simulink model "part2_MAIN"  (R2023b)
settings: Solver=FixedStepAuto  StartTime=0.0  StopTime=300  FixedStep=0.1  RelTol=1e-3
values from neighbouring files (symbols this model uses):
  Af = diag(ti)    [init.m]
  Aw = [zeros(3) eye(3) ... (first row only)    [get_observer_parameters.m]
  B = [zeros(6,3);zeros(3,3);zeros(3,3);inv(M)]    [get_observer_parameters.m]
  change_position_time = 1200    [init.m]
  Cw = [zeros(3) eye(3)]    [get_observer_parameters.m]
  D = Damping    [init.m]
  Damping = diag([2.6486e5, 8.8164e5, 3.3774e8])    [init.m]
  direction_limit = pi/36    (= 0.0872664625997)    [init.m]
  direction_time_constant = 100    [init.m]
  dt = 0.1    [get_observer_parameters.m]
  E = [Ew, zeros(6,3) ... (first row only)    [get_observer_parameters.m]
  Gamma = diag(omega_is)    [init.m]
  gust_limit = 40    [init.m]
  H = [Cw, eye(3), zeros(3,3) zeros(3,3)]    [get_observer_parameters.m]
  height = 3    [init.m]
  inv_M = inv(M)    [get_observer_parameters.m]
  inv_Tb = inv(Tb)    [get_observer_parameters.m]
  kappa = 0.003    [init.m]
  kappa2 = 0.0026    [init.m]
  Kd = [1660451.40544401; 3920391.80535684; 1605063439.04156]    [init.m]
  Ki = [137.081306245593; 3163.274947400198; 335358.448218978]    [init.m]
  Kp = [75459.3345349083; 277551.73586971; 120744473.878042]    [init.m]
  L = 1800    [init.m]
  M = Mass    [init.m]
  mean_wind_direction = pi    (= 3.14159265359)    [init.m]
  observer_type = 0    [init.m]
  Omega = diag([omega_n])    [get_observer_parameters.m]    (also in init.m = diag(2*omega_is.*zeta_is))
  Q = diag([0.1,0.1,pi/180,1e6,1e6,1e9])*10e3    [get_observer_parameters.m]
  R = diag([0.00001,0.00001,0.01*pi/180])*10e-4    [get_observer_parameters.m]
  simu_step = 36    [init.m]
  simulation = 5    [init.m]
  slow_varying_limit = 1    [init.m]
  slow_varying_time_constant = 100    [init.m]
  TAU = dt*E    [get_observer_parameters.m]
  Tb = 0.1 * eye(3)    [get_observer_parameters.m]
  thruster_type = 0    [init.m]
  u10 = 12    [init.m]
  wind = 1    [init.m]
  x_current = u_c*cos(xi)    [init.m]
  y_current = u_c*sin(xi)    [init.m]
undefined symbols (not defined in the file or in its folder): Hoerner, ModelParams, npf, Param, thrusters, vessel, WaveModel
libraries: dspsigops x42, simulink x30, marine_hydro x16, marine_gnc x8, slpidlib x3
(part 3 of 8)

== system part2_MAIN/Simulation 4/Wave ==
  eta : Inport
  waves : Inport  Port=2
  Gain : Gain  Gain=waveforces
  Sum : Sum
  Wave loads (U=0) : marine_hydro/Hydro Library/Wave loads (U=0)  SystemSampleTime=-1  VariantActivationTime=update diagram  AllowFlexibleInterface=on  Latency=0  AutoFrameSizeCalculation=off
  Wave : Outport  VectorParamsAs1DForOutWhenUnconnected=off
  wires:
  eta/1 -> Wave loads (U=0)/1
  waves/1 -> Wave loads (U=0)/2
  Sum/1 -> Gain/1
  Wave loads (U=0)/1 -> Sum/1
  Wave loads (U=0)/2 -> Sum/2
  Gain/1 -> Wave/1

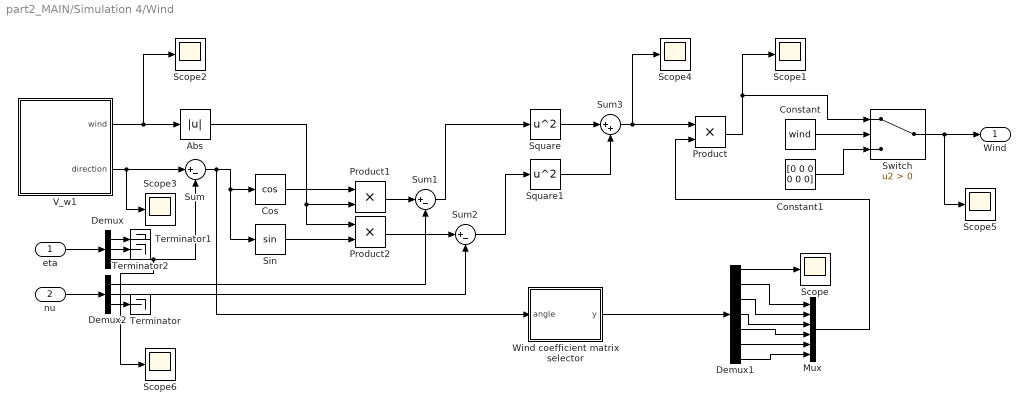
== system part2_MAIN/Simulation 4/Wind ==
  eta : Inport
  nu : Inport  Port=2
  Abs : Abs  SaturateOnIntegerOverflow=off
  Constant : Constant  Value=wind
  Constant1 : Constant  Value=[0 0 0 0 0 0]
  Cos : Trigonometry  Operator=cos
  Demux : Demux  Outputs=3
  Demux1 : Demux  Outputs=7
  Demux2 : Demux  Outputs=3
  Mux : Mux  Inputs=6
  Product : Product
  Product1 : Product
  Product2 : Product
  Scope{,1..6} (7 alike) : Scope
  Sin : Trigonometry
  Square : Math  Operator=square  SignedPower=on
  Square1 : Math  Operator=square  SignedPower=on
  Sum : Sum  Inputs=|+-
  Sum1 : Sum  Inputs=|+-
  Sum2 : Sum  Inputs=|+-
  Sum3 : Sum  Inputs=|++
  Switch : Switch  Criteria=u2 > Threshold  SaturateOnIntegerOverflow=off  InputSameDT=off
  Terminator : Terminator
  Terminator1 : Terminator
  Terminator2 : Terminator
  V_w1 : Subsystem
  Wind coefficient matrix selector : MATLAB Function  TreatAsAtomicUnit=on
  Wind : Outport  VectorParamsAs1DForOutWhenUnconnected=off
  wires:
  V_w1/1(wind) -> Scope2/1, Abs/1
  Abs/1 -> Product2/1, Product1/2
  eta/1 -> Demux/1
  V_w1/2(direction) -> Scope3/1, Sum/1
  Demux/3 -> Scope6/1, Sum/2
  Wind coefficient matrix selector/1(y) -> Demux1/1
  Demux1/1 -> Scope/1
  Demux1/2 -> Mux/1
  Demux1/3 -> Mux/2
  Demux1/4 -> Mux/3
  Demux1/5 -> Mux/4
  Demux1/6 -> Mux/5
  Demux1/7 -> Mux/6
  Product/1 -> Switch/1, Scope1/1
  Mux/1 -> Product/2
  Sum/1 -> Wind coefficient matrix selector/1(angle), Sin/1, Cos/1
  nu/1 -> Demux2/1
  Sin/1 -> Product2/2
  Cos/1 -> Product1/1
  Product1/1 -> Sum1/1
  Product2/1 -> Sum2/1
  Demux2/1 -> Sum1/2
  Demux2/2 -> Sum2/2
  Sum1/1 -> Square/1
  Sum2/1 -> Square1/1
  Sum3/1 -> Scope4/1, Product/1
  Square/1 -> Sum3/1
  Square1/1 -> Sum3/2
  Demux2/3 -> Terminator/1
  Demux/1 -> Terminator1/1
  Demux/2 -> Terminator2/1
  Switch/1 -> Scope5/1, Wind/1
  Constant/1 -> Switch/2
  Constant1/1 -> Switch/3

== system part2_MAIN/Simulation 5/Current (North - East) ==
  note: simulation 2
  note: simulation 1
  eta : Inport
  Constant : Constant
  Constant1 : Constant  Value=[0.5*cos(135); 0.5*sin(135); 0]
  Demux : Demux  Outputs=3
  MATLAB Function : MATLAB Function  TreatAsAtomicUnit=on
  Matrix Multiply : Product  Multiplication=Matrix(*)
  Mux : Mux
  Scope : Scope  NumInputPorts=2
  Scope1 : Scope
  Step : Step  After=0  SampleTime=0
  Subsystem : Subsystem
  Subsystem1 : Subsystem
  Subsystem2 : Subsystem
  Switch : Switch  Criteria=u2 > Threshold  Threshold=1  SaturateOnIntegerOverflow=off  InputSameDT=off
  Switch1 : Switch  Criteria=u2 > Threshold  Threshold=2  SaturateOnIntegerOverflow=off  InputSameDT=off
  Terminator : Terminator
  Terminator1 : Terminator
  Terminator2 : Terminator
  To Workspace : ToWorkspace  VariableName=Current  SaveFormat=Timeseries  SampleTime=-1
  Current1 : Outport  VectorParamsAs1DForOutWhenUnconnected=off
  wires:
  Demux/2 -> Terminator1/1
  MATLAB Function/1(y) -> Matrix Multiply/1
  Switch/1 -> Switch1/3
  Matrix Multiply/1 -> Scope/2, Mux/1
  Subsystem2/1(Out1) -> Switch1/1
  Subsystem/1(Out1) -> Switch/3
  Subsystem1/1(Out1) -> Switch/1
  Demux/1 -> Terminator/1
  Switch1/1 -> Scope/1, To Workspace/1, Matrix Multiply/2
  eta/1 -> Demux/1  "eta"
  Constant/1 -> Switch1/2, Switch/2
  Constant1/1 -> Terminator2/1
  Step/1 -> Mux/3, Mux/2, Mux/4
  Demux/3 -> MATLAB Function/1(u)
  Mux/1 -> Scope1/1, Current1/1

== system part2_MAIN/Simulation 5/DP Controller ==
  note: PID controller
  note: Velocity
  note: Position
  nu : Inport
  eta : Inport  Port=2
  eta set point : Inport  Port=3
  nu setpoint : Inport  Port=4
  Add : Sum  Inputs=+++
  Constant : Constant  Value=0
  Demux{,1,3..4} (4 alike) : Demux  Outputs=3
  Gain : Gain  Gain=Kd
  Gain1 : Gain  Gain=Kp
  Gain2 : Gain  Gain=Ki
  Integrator : Integrator
  MATLAB Function : MATLAB Function  TreatAsAtomicUnit=on
  MATLAB Function1 : MATLAB Function  TreatAsAtomicUnit=on
  Matrix Multiply : Product  Multiplication=Matrix(*)
  Matrix Multiply1 : Product  Multiplication=Matrix(*)
  Mux : Mux  Inputs=3
  Mux2 : Mux  Inputs=6
  Mux3 : Mux  Inputs=3
  Scope : Scope
  Step : Step  After=0  SampleTime=0
  Sum{,1..3} (4 alike) : Sum  Inputs=|-+
  Terminator1 : Terminator
  To Workspace : ToWorkspace  VariableName=simout2  SaveFormat=Timeseries  SampleTime=-1
  tau (body frame) : Outport  VectorParamsAs1DForOutWhenUnconnected=off
  wires:
  eta/1 -> Demux/1  "eta"
  eta set point/1 -> Demux1/1
  Demux/1 -> Sum2/1  "n_vessel"
  Demux1/1 -> Sum2/2  "n_sp"
  Demux/2 -> Sum/1  "e_vessel"
  Demux1/2 -> Sum/2  "e_sp"
  Sum2/1 -> Mux/1
  Sum/1 -> Mux/2
  MATLAB Function/1(y) -> Matrix Multiply/1
  Mux/1 -> Matrix Multiply/2  "error NED frame"
  Step/1 -> Mux2/4, Mux2/3, Mux2/5
  Demux1/3 -> Sum1/2, MATLAB Function1/1(u)  "yaw_sp"
  Sum1/1 -> Mux3/3
  Constant/1 -> Mux/3
  Demux/3 -> MATLAB Function/1(u), Sum1/1  "yaw_vessel"
  Matrix Multiply/1 -> Demux4/1  "error body frame"
  nu/1 -> Sum3/1
  Sum3/1 -> Gain/1  "error body frame"
  nu setpoint/1 -> Matrix Multiply1/2
  MATLAB Function1/1(y) -> Matrix Multiply1/1
  Matrix Multiply1/1 -> Sum3/2
  Integrator/1 -> Gain2/1
  Gain1/1 -> Add/1
  Gain2/1 -> Add/2
  Gain/1 -> Add/3
  Demux3/1 -> Mux2/1
  Demux3/2 -> Mux2/2
  Demux3/3 -> Mux2/6
  Demux4/1 -> Mux3/1
  Demux4/2 -> Mux3/2
  Demux4/3 -> Terminator1/1
  Mux3/1 -> Integrator/1, Gain1/1
  Mux2/1 -> tau (body frame)/1
  Add/1 -> To Workspace/1, Scope/1, Demux3/1

== system part2_MAIN/Simulation 5/Observer ==
  y : Inport
  tau_est : Inport  Port=2
  Demux : Demux  Outputs=2
  EKF : Subsystem
  Memory : Memory  InitialCondition=zeros(3,1)
  Memory2 : Memory  InitialCondition=zeros(3,1)
  Mux : Mux  Inputs=2
  Mux1 : Mux  Inputs=2
  Observer Selector : Constant  Value=observer_type
  Passive Non-Linear : Subsystem
  Subsystem : Subsystem
  Switch : Switch  Criteria=u2 > Threshold  SaturateOnIntegerOverflow=off  InputSameDT=off
  nu_hat : Outport  VectorParamsAs1DForOutWhenUnconnected=off
  eta_hat : Outport  Port=2  VectorParamsAs1DForOutWhenUnconnected=off
  wires:
  tau_est/1 -> Subsystem/1(In1)
  Memory/1 -> EKF/2(U)
  Subsystem/1(Out1) -> Memory/1, Memory2/1
  EKF/1(eta_hat) -> Mux/1
  EKF/2(nu_hat) -> Mux/2
  Passive Non-Linear/1(eta_hat) -> Mux1/1
  Passive Non-Linear/2(nu_hat) -> Mux1/2
  Mux1/1 -> Switch/1
  Observer Selector/1 -> Switch/2
  Mux/1 -> Switch/3
  Switch/1 -> Demux/1
  Demux/1 -> eta_hat/1
  Demux/2 -> nu_hat/1
  y/1 -> EKF/1(y), Passive Non-Linear/1(y)
  Memory2/1 -> Passive Non-Linear/2(tau_est)

== system part2_MAIN/Simulation 5/Reference Model ==
  note: Af
  note: eta_r
  note: Xref
  note: omega
  note: eta_r - Xref
  note: Gamma
  note: x_ddot
  note: Gamma
  note: X_dot
  note: X
  Add : Sum  Inputs=+--
  Gain : Gain  Gain=Af  Multiplication=Matrix(K*u)
  Gain1 : Gain  Gain=Gamma  Multiplication=Matrix(K*u)
  Gain2 : Gain  Gain=Omega  Multiplication=Matrix(K*u)
  Gain3 : Gain  Gain=Gamma  Multiplication=Matrix(K*u)
  Integrator : Integrator
  Integrator1 : Integrator
  Integrator2 : Integrator
  Scope : Scope  NumInputPorts=2
  Scope1 : Scope
  Scope2 : Scope
  Simulation Selector : Subsystem
  Sum : Sum  Inputs=|+-
  To Workspace : ToWorkspace  VariableName=Reference  SaveFormat=Timeseries  SampleTime=-1
  Set-point : Outport  VectorParamsAs1DForOutWhenUnconnected=off
  nu set point : Outport  Port=2  VectorParamsAs1DForOutWhenUnconnected=off
  wires:
  Integrator/1 -> Gain1/1, Sum/2
  Add/1 -> Scope2/1, Integrator1/1
  Integrator2/1 -> To Workspace/1, Scope/1, Set-point/1, Gain3/1
  Gain1/1 -> Add/1
  Integrator1/1 -> nu set point/1, Scope/2, Integrator2/1, Gain2/1
  Gain/1 -> Integrator/1
  Gain2/1 -> Add/3
  Gain3/1 -> Add/2
  Simulation Selector/1(Out1) -> Scope1/1, Sum/1
  Sum/1 -> Gain/1

== system part2_MAIN/Simulation 5/Thrust Allocation ==
  tau_d : Inport
  0 : MATLAB Function  TreatAsAtomicUnit=on
  1 : MATLAB Function  Commented=on  TreatAsAtomicUnit=on
  Constant : Constant  Value=thruster_type
  Switch : Switch  Criteria=u2 > Threshold  SaturateOnIntegerOverflow=off  InputSameDT=off
  Switch1 : Switch  Criteria=u2 > Threshold  SaturateOnIntegerOverflow=off  InputSameDT=off
  Unwrap : Subsystem
  Unwrap1 : Subsystem
  u : Outport  VectorParamsAs1DForOutWhenUnconnected=off
  alpha [rad] : Outport  Port=2  VectorParamsAs1DForOutWhenUnconnected=off
  wires:
  tau_d/1 -> 1/1(tau_d), 0/1(tau_d)
  1/2(alpha) -> Unwrap/1(alpha)
  0/2(alpha) -> Unwrap1/1(alpha)
  1/1(Td) -> Switch/1
  Constant/1 -> Switch1/2, Switch/2
  0/1(Td) -> Switch/3
  Unwrap/1(alpha [rad]) -> Switch1/1
  Unwrap1/1(alpha [rad]) -> Switch1/3
  Switch/1 -> u/1
  Switch1/1 -> alpha [rad]/1

== system part2_MAIN/Simulation 5/Thruster Dynamics ==
  u [N] : Inport
  alpha [rad] : Inport  Port=2
  Constant : Constant  Value=[thrusters(1).xposition, thrusters(2).xposition, thrusters(3).xposition, thrusters(4).xposition, thrusters(5).xposition]
  Constant1 : Constant  Value=zeros(3,1)
  Constant2 : Constant  Value=[thrusters(1).yposition, thrusters(2).yposition, thrusters(3).yposition, thrusters(4).yposition, thrusters(5).yposition]
  Demux : Demux  Outputs=5
  Demux1 : Demux  Outputs=5
  Gain1 : Gain  Gain=1-thrusterfault
  Gain2 : Gain  Gain=1-thrusterfault
  MATLAB Function : MATLAB Function  TreatAsAtomicUnit=on
  Mux1 : Mux  Inputs=2
  Rate Limiter : RateLimiter  RisingSlewLimit=thrusters(1).rate  FallingSlewLimit=-thrusters(1).rate  SampleTimeMode=inherited
  Rate Limiter1 : RateLimiter  RisingSlewLimit=thrusters(2).rate  FallingSlewLimit=-thrusters(2).rate  SampleTimeMode=inherited
  Rate Limiter10 : RateLimiter  RisingSlewLimit=thrusters(4).rotationspeed  FallingSlewLimit=-thrusters(4).rotationspeed  SampleTimeMode=inherited
  Rate Limiter11 : RateLimiter  RisingSlewLimit=thrusters(5).rotationspeed  FallingSlewLimit=-thrusters(5).rotationspeed  SampleTimeMode=inherited
  Rate Limiter2 : RateLimiter  RisingSlewLimit=thrusters(3).rate  FallingSlewLimit=-thrusters(3).rate  SampleTimeMode=inherited
  Rate Limiter4 : RateLimiter  RisingSlewLimit=thrusters(4).rate  FallingSlewLimit=-thrusters(4).rate  SampleTimeMode=inherited
  Rate Limiter5 : RateLimiter  RisingSlewLimit=thrusters(5).rate  FallingSlewLimit=-thrusters(5).rate  SampleTimeMode=inherited
  Rate Limiter8 : RateLimiter  RisingSlewLimit=thrusters(2).rotationspeed  FallingSlewLimit=-thrusters(2).rotationspeed  SampleTimeMode=inherited
  Saturation : Saturate  UpperLimit=thrusters(1).thrust  LowerLimit=-thrusters(1).thrust
  Saturation1 : Saturate  UpperLimit=thrusters(2).thrust  LowerLimit=-thrusters(2).thrust
  Saturation2 : Saturate  UpperLimit=thrusters(3).thrust  LowerLimit=-thrusters(3).thrust
  Saturation4 : Saturate  UpperLimit=thrusters(4).thrust  LowerLimit=-thrusters(4).thrust
  Saturation5 : Saturate  UpperLimit=thrusters(5).thrust  LowerLimit=-thrusters(5).thrust
  Selector4 : Selector  InputPortWidth=6  IndexOptions=Index vector (dialog)  Indices=[1 2 4 5 6 3]  OutputSizes=1
  alpha : Mux  Inputs=5
  u : Mux  Inputs=5
  "Forces (body frame) " : Outport  VectorParamsAs1DForOutWhenUnconnected=off
  wires:
  Rate Limiter2/1 -> u/3
  Saturation/1 -> Rate Limiter/1
  Mux1/1 -> Selector4/1
  Constant1/1 -> Mux1/2
  Saturation4/1 -> Rate Limiter4/1
  Demux/2 -> Saturation1/1
  Saturation1/1 -> Rate Limiter1/1
  Demux/1 -> Saturation/1
  Demux/3 -> Saturation2/1
  Saturation2/1 -> Rate Limiter2/1
  Selector4/1 -> "Forces (body frame) "/1
  Gain1/1 -> u/2
  Rate Limiter1/1 -> Gain1/1
  Rate Limiter/1 -> u/1
  Rate Limiter4/1 -> Gain2/1
  Saturation5/1 -> Rate Limiter5/1
  u [N]/1 -> Demux/1
  alpha [rad]/1 -> Demux1/1
  Constant/1 -> MATLAB Function/3(PosX)
  Constant2/1 -> MATLAB Function/4(PosY)
  u/1 -> MATLAB Function/2(thrust_actual)
  alpha/1 -> MATLAB Function/1(alpha_actual)
  MATLAB Function/1(actual_tau) -> Mux1/1
  Rate Limiter10/1 -> alpha/4
  Demux1/4 -> Rate Limiter10/1
  Demux1/5 -> Rate Limiter11/1
  Rate Limiter11/1 -> alpha/5
  Demux1/1 -> alpha/1
  Gain2/1 -> u/4
  Demux/4 -> Saturation4/1
  Demux/5 -> Saturation5/1
  Rate Limiter5/1 -> u/5
  Demux1/2 -> Rate Limiter8/1
  Rate Limiter8/1 -> alpha/2
  Demux1/3 -> alpha/3

== system part2_MAIN/Simulation 5/Wave ==
  eta : Inport
  waves : Inport  Port=2
  Gain : Gain  Gain=waveforces
  Sum : Sum
  Wave loads (U=0) : marine_hydro/Hydro Library/Wave loads (U=0)  SystemSampleTime=-1  VariantActivationTime=update diagram  AllowFlexibleInterface=on  Latency=0  AutoFrameSizeCalculation=off
  Wave : Outport  VectorParamsAs1DForOutWhenUnconnected=off
  wires:
  eta/1 -> Wave loads (U=0)/1
  waves/1 -> Wave loads (U=0)/2
  Sum/1 -> Gain/1
  Wave loads (U=0)/1 -> Sum/1
  Wave loads (U=0)/2 -> Sum/2
  Gain/1 -> Wave/1

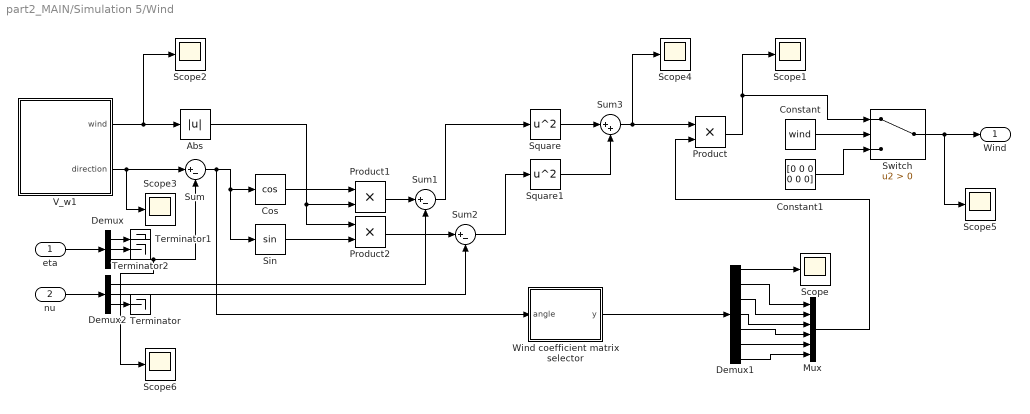
== system part2_MAIN/Simulation 5/Wind ==
  eta : Inport
  nu : Inport  Port=2
  Abs : Abs  SaturateOnIntegerOverflow=off
  Constant : Constant  Value=wind
  Constant1 : Constant  Value=[0 0 0 0 0 0]
  Cos : Trigonometry  Operator=cos
  Demux : Demux  Outputs=3
  Demux1 : Demux  Outputs=7
  Demux2 : Demux  Outputs=3
  Mux : Mux  Inputs=6
  Product : Product
  Product1 : Product
  Product2 : Product
  Scope{,1..6} (7 alike) : Scope
  Sin : Trigonometry
  Square : Math  Operator=square  SignedPower=on
  Square1 : Math  Operator=square  SignedPower=on
  Sum : Sum  Inputs=|+-
  Sum1 : Sum  Inputs=|+-
  Sum2 : Sum  Inputs=|+-
  Sum3 : Sum  Inputs=|++
  Switch : Switch  Criteria=u2 > Threshold  SaturateOnIntegerOverflow=off  InputSameDT=off
  Terminator : Terminator
  Terminator1 : Terminator
  Terminator2 : Terminator
  V_w1 : Subsystem
  Wind coefficient matrix selector : MATLAB Function  TreatAsAtomicUnit=on
  Wind : Outport  VectorParamsAs1DForOutWhenUnconnected=off
  wires:
  V_w1/1(wind) -> Scope2/1, Abs/1
  Abs/1 -> Product2/1, Product1/2
  eta/1 -> Demux/1
  V_w1/2(direction) -> Scope3/1, Sum/1
  Demux/3 -> Scope6/1, Sum/2
  Wind coefficient matrix selector/1(y) -> Demux1/1
  Demux1/1 -> Scope/1
  Demux1/2 -> Mux/1
  Demux1/3 -> Mux/2
  Demux1/4 -> Mux/3
  Demux1/5 -> Mux/4
  Demux1/6 -> Mux/5
  Demux1/7 -> Mux/6
  Product/1 -> Switch/1, Scope1/1
  Mux/1 -> Product/2
  Sum/1 -> Wind coefficient matrix selector/1(angle), Sin/1, Cos/1
  nu/1 -> Demux2/1
  Sin/1 -> Product2/2
  Cos/1 -> Product1/1
  Product1/1 -> Sum1/1
  Product2/1 -> Sum2/1
  Demux2/1 -> Sum1/2
  Demux2/2 -> Sum2/2
  Sum1/1 -> Square/1
  Sum2/1 -> Square1/1
  Sum3/1 -> Scope4/1, Product/1
  Square/1 -> Sum3/1
  Square1/1 -> Sum3/2
  Demux2/3 -> Terminator/1
  Demux/1 -> Terminator1/1
  Demux/2 -> Terminator2/1
  Switch/1 -> Scope5/1, Wind/1
  Constant/1 -> Switch/2
  Constant1/1 -> Switch/3

== system part2_MAIN/Simulation 6/Current (North - East) ==
  note: simulation 2
  note: simulation 1
  eta : Inport
  Constant1 : Constant  Value=[0.5*cos(135); 0.5*sin(135); 0]
  Demux : Demux  Outputs=3
  MATLAB Function : MATLAB Function  TreatAsAtomicUnit=on
  Matrix Multiply : Product  Multiplication=Matrix(*)
  Mux : Mux
  Scope : Scope  NumInputPorts=2
  Scope1 : Scope
  Step : Step  After=0  SampleTime=0
  Subsystem : Subsystem
  Terminator : Terminator
  Terminator1 : Terminator
  Terminator2 : Terminator
  To Workspace : ToWorkspace  VariableName=Current  SaveFormat=Timeseries  SampleTime=-1
  Current1 : Outport  VectorParamsAs1DForOutWhenUnconnected=off
  wires:
  Demux/2 -> Terminator1/1
  MATLAB Function/1(y) -> Matrix Multiply/1
  Matrix Multiply/1 -> Scope/2, Mux/1
  Demux/1 -> Terminator/1
  Subsystem/1(Out1) -> Scope/1, To Workspace/1, Matrix Multiply/2
  eta/1 -> Demux/1  "eta"
  Constant1/1 -> Terminator2/1
  Step/1 -> Mux/3, Mux/2, Mux/4
  Demux/3 -> MATLAB Function/1(u)
  Mux/1 -> Scope1/1, Current1/1

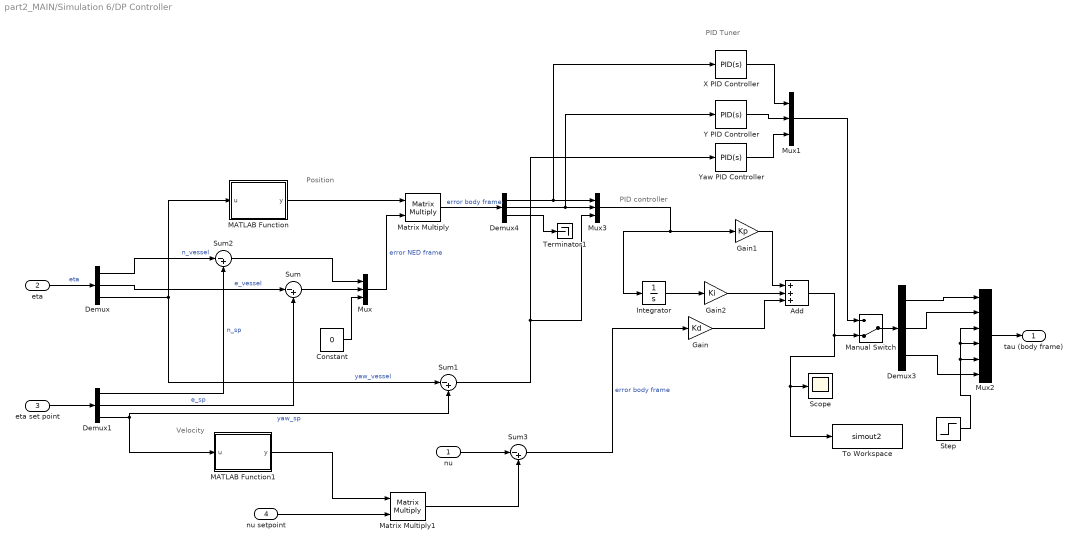
== system part2_MAIN/Simulation 6/DP Controller ==
  note: PID Tuner
  note: PID controller
  note: Velocity
  note: Position
  nu : Inport
  eta : Inport  Port=2
  eta set point : Inport  Port=3
  nu setpoint : Inport  Port=4
  Add : Sum  Inputs=+++
  Constant : Constant  Value=0
  Demux{,1,3..4} (4 alike) : Demux  Outputs=3
  Gain : Gain  Gain=Kd
  Gain1 : Gain  Gain=Kp
  Gain2 : Gain  Gain=Ki
  Integrator : Integrator
  MATLAB Function : MATLAB Function  TreatAsAtomicUnit=on
  MATLAB Function1 : MATLAB Function  TreatAsAtomicUnit=on
  Manual Switch : ManualSwitch  CurrentSetting=0
  Matrix Multiply : Product  Multiplication=Matrix(*)
  Matrix Multiply1 : Product  Multiplication=Matrix(*)
  Mux : Mux  Inputs=3
  Mux1 : Mux  Inputs=3
  Mux2 : Mux  Inputs=6
  Mux3 : Mux  Inputs=3
  Scope : Scope
  Step : Step  After=0  SampleTime=0
  Sum{,1..3} (4 alike) : Sum  Inputs=|-+
  Terminator1 : Terminator
  To Workspace : ToWorkspace  VariableName=simout2  SaveFormat=Timeseries  SampleTime=-1
  X PID Controller : slpidlib/PID Controller  Controller=PID  Form=Parallel  TimeDomain=Continuous-time  UseExternalTs=off  SampleTime=-1  IntegratorMethod=Forward Euler  FilterMethod=Forward Euler  ControllerParametersSource=internal  P=68459.3345349083  I=80.081306245593  UseKiTs=off  D=1660451.40544401  N=0.143790431530358  UseFilter=on  TunerSelectOption=Transfer Function Based (PID Tuner App)  InitialConditionSource=internal  InitialConditionForIntegrator=0  InitialConditionForFilter=0  DifferentiatorICPrevScaledInput=0  ExternalReset=none  TrackingMode=off  Kt=1  LimitOutput=off  SatLimitsSource=internal  UpperSaturationLimit=inf  LowerSaturationLimit=-inf  LinearizeAsGain=on  AntiWindupMode=none  Kb=1  LimitIntegrator=off  UpperIntegratorSaturationLimit=inf  LowerIntegratorSaturationLimit=-inf  POutMin=[]  POutMax=[]  IOutMin=[]  IOutMax=[]  DOutMin=[]  DOutMax=[]  NOutMin=[]  NOutMax=[]  SumOutMin=[]  SumOutMax=[]  SaturationOutMin=[]  SaturationOutMax=[]  PParamMin=[]  PParamMax=[]  IParamMin=[]  IParamMax=[]  DParamMin=[]  DParamMax=[]  NParamMin=[]  NParamMax=[]  KbParamMin=[]  KbParamMax=[]  KtParamMin=[]  KtParamMax=[]  KbOutMin=[]  KbOutMax=[]  KtOutMin=[]  KtOutMax=[]  IntegratorOutMin=[]  IntegratorOutMax=[]  FilterOutMin=[]  FilterOutMax=[]  SumI1OutMin=[]  SumI1OutMax=[]  SumI2OutMin=[]  SumI2OutMax=[]  SumI3OutMin=[]  SumI3OutMax=[]  SumI4OutMin=[]  SumI4OutMax=[]  SumDOutMin=[]  SumDOutMax=[]  DifferentiatorOutMin=[]  DifferentiatorOutMax=[]  FilterDiffOutCoefMin=[]  FilterDiffOutCoefMax=[]  ReciprocalOutMin=[]  ReciprocalOutMax=[]  SumDenOutMin=[]  SumDenOutMax=[]  SumNumOutMin=[]  SumNumOutMax=[]  DivideOutMin=[]  DivideOutMax=[]  UdiffTsProdOutMin=[]  UdiffTsProdOutMax=[]  NTsProdOutMin=[]  NTsProdOutMax=[]  UintegralTsProdOutMin=[]  UintegralTsProdOutMax=[]  UngainTsProdOutMin=[]  UngainTsProdOutMax=[]  ClampingZeroOutDataTypeStr=Inherit: Inherit via back propagation  ClampingZeroOutMin=[]  ClampingZeroOutMax=[]  FilterDenConstantOutDataTypeStr=Inherit: Inherit via back propagation  FilterDenConstantOutMin=[]  FilterDenConstantOutMax=[]  PCopyOutDataTypeStr=Inherit: Inherit via back propagation  PCopyOutMin=[]  PCopyOutMax=[]  NCopyOutDataTypeStr=Inherit: Inherit via back propagation  NCopyOutMin=[]  NCopyOutMax=[]  IntegratorContinuousStateAttributes=''  IntegratorStateMustResolveToSignalObject=off  IntegratorRTWStateStorageClass=Auto  FilterContinuousStateAttributes=''  FilterStateMustResolveToSignalObject=off  FilterRTWStateStorageClass=Auto  ParallelPVariant=InternalParameters  IdealPVariant=Disabled  IVariant=InternalParameters  DVariant=InternalParameters  IntegratorVariant=Continuous  SatVariant=Disabled  AWVariant=Passthrough  PCopyVariant=Disabled  TRVariant=Disabled  FdbkBlocksVariant=Forward  IdealPFdbkVariant=Disabled  SatFdbkVariant=Disabled  DerivativeFilterVariant=ContFilter  NVariant=InternalParameters  NCopyVariant=Disabled  FilterICVariant=InternalICsFilter  IntegratorICVariant=InternalICs  ExternalResetVariant=Disabled  TRSumVariant=Passthrough  SumFdbkVariant=Disabled  SumVariant=Sum_PID  TsampFilterVariant=InternalTs  TsampNgainVariant=Passthrough  TsampIntegralVariant=Disabled_SignalSpec  ExternalSaturationOutDataTypeStr=Inherit: Same as second input
  Y PID Controller : slpidlib/PID Controller  Controller=PID  Form=Parallel  TimeDomain=Continuous-time  UseExternalTs=off  SampleTime=-1  IntegratorMethod=Forward Euler  FilterMethod=Forward Euler  ControllerParametersSource=internal  P=377551.73586971  I=863.274947400198  UseKiTs=off  D=3920391.80535684  N=9.58373501278933  UseFilter=on  TunerSelectOption=Transfer Function Based (PID Tuner App)  InitialConditionSource=internal  InitialConditionForIntegrator=0  InitialConditionForFilter=0  DifferentiatorICPrevScaledInput=0  ExternalReset=none  TrackingMode=off  Kt=1  LimitOutput=off  SatLimitsSource=internal  UpperSaturationLimit=inf  LowerSaturationLimit=-inf  LinearizeAsGain=on  AntiWindupMode=none  Kb=1  LimitIntegrator=off  UpperIntegratorSaturationLimit=inf  LowerIntegratorSaturationLimit=-inf  POutMin=[]  POutMax=[]  IOutMin=[]  IOutMax=[]  DOutMin=[]  DOutMax=[]  NOutMin=[]  NOutMax=[]  SumOutMin=[]  SumOutMax=[]  SaturationOutMin=[]  SaturationOutMax=[]  PParamMin=[]  PParamMax=[]  IParamMin=[]  IParamMax=[]  DParamMin=[]  DParamMax=[]  NParamMin=[]  NParamMax=[]  KbParamMin=[]  KbParamMax=[]  KtParamMin=[]  KtParamMax=[]  KbOutMin=[]  KbOutMax=[]  KtOutMin=[]  KtOutMax=[]  IntegratorOutMin=[]  IntegratorOutMax=[]  FilterOutMin=[]  FilterOutMax=[]  SumI1OutMin=[]  SumI1OutMax=[]  SumI2OutMin=[]  SumI2OutMax=[]  SumI3OutMin=[]  SumI3OutMax=[]  SumI4OutMin=[]  SumI4OutMax=[]  SumDOutMin=[]  SumDOutMax=[]  DifferentiatorOutMin=[]  DifferentiatorOutMax=[]  FilterDiffOutCoefMin=[]  FilterDiffOutCoefMax=[]  ReciprocalOutMin=[]  ReciprocalOutMax=[]  SumDenOutMin=[]  SumDenOutMax=[]  SumNumOutMin=[]  SumNumOutMax=[]  DivideOutMin=[]  DivideOutMax=[]  UdiffTsProdOutMin=[]  UdiffTsProdOutMax=[]  NTsProdOutMin=[]  NTsProdOutMax=[]  UintegralTsProdOutMin=[]  UintegralTsProdOutMax=[]  UngainTsProdOutMin=[]  UngainTsProdOutMax=[]  ClampingZeroOutDataTypeStr=Inherit: Inherit via back propagation  ClampingZeroOutMin=[]  ClampingZeroOutMax=[]  FilterDenConstantOutDataTypeStr=Inherit: Inherit via back propagation  FilterDenConstantOutMin=[]  FilterDenConstantOutMax=[]  PCopyOutDataTypeStr=Inherit: Inherit via back propagation  PCopyOutMin=[]  PCopyOutMax=[]  NCopyOutDataTypeStr=Inherit: Inherit via back propagation  NCopyOutMin=[]  NCopyOutMax=[]  IntegratorContinuousStateAttributes=''  IntegratorStateMustResolveToSignalObject=off  IntegratorRTWStateStorageClass=Auto  FilterContinuousStateAttributes=''  FilterStateMustResolveToSignalObject=off  FilterRTWStateStorageClass=Auto  ParallelPVariant=InternalParameters  IdealPVariant=Disabled  IVariant=InternalParameters  DVariant=InternalParameters  IntegratorVariant=Continuous  SatVariant=Disabled  AWVariant=Passthrough  PCopyVariant=Disabled  TRVariant=Disabled  FdbkBlocksVariant=Forward  IdealPFdbkVariant=Disabled  SatFdbkVariant=Disabled  DerivativeFilterVariant=ContFilter  NVariant=InternalParameters  NCopyVariant=Disabled  FilterICVariant=InternalICsFilter  IntegratorICVariant=InternalICs  ExternalResetVariant=Disabled  TRSumVariant=Passthrough  SumFdbkVariant=Disabled  SumVariant=Sum_PID  TsampFilterVariant=InternalTs  TsampNgainVariant=Passthrough  TsampIntegralVariant=Disabled_SignalSpec  ExternalSaturationOutDataTypeStr=Inherit: Same as second input
  Yaw PID Controller : slpidlib/PID Controller  Controller=PID  Form=Parallel  TimeDomain=Continuous-time  UseExternalTs=off  SampleTime=-1  IntegratorMethod=Forward Euler  FilterMethod=Forward Euler  ControllerParametersSource=internal  P=120744473.878042  I=335358.448218978  UseKiTs=off  D=1605063439.04156  N=0.143717056319525  UseFilter=on  TunerSelectOption=Transfer Function Based (PID Tuner App)  InitialConditionSource=internal  InitialConditionForIntegrator=0  InitialConditionForFilter=0  DifferentiatorICPrevScaledInput=0  ExternalReset=none  TrackingMode=off  Kt=1  LimitOutput=off  SatLimitsSource=internal  UpperSaturationLimit=inf  LowerSaturationLimit=-inf  LinearizeAsGain=on  AntiWindupMode=none  Kb=1  LimitIntegrator=off  UpperIntegratorSaturationLimit=inf  LowerIntegratorSaturationLimit=-inf  POutMin=[]  POutMax=[]  IOutMin=[]  IOutMax=[]  DOutMin=[]  DOutMax=[]  NOutMin=[]  NOutMax=[]  SumOutMin=[]  SumOutMax=[]  SaturationOutMin=[]  SaturationOutMax=[]  PParamMin=[]  PParamMax=[]  IParamMin=[]  IParamMax=[]  DParamMin=[]  DParamMax=[]  NParamMin=[]  NParamMax=[]  KbParamMin=[]  KbParamMax=[]  KtParamMin=[]  KtParamMax=[]  KbOutMin=[]  KbOutMax=[]  KtOutMin=[]  KtOutMax=[]  IntegratorOutMin=[]  IntegratorOutMax=[]  FilterOutMin=[]  FilterOutMax=[]  SumI1OutMin=[]  SumI1OutMax=[]  SumI2OutMin=[]  SumI2OutMax=[]  SumI3OutMin=[]  SumI3OutMax=[]  SumI4OutMin=[]  SumI4OutMax=[]  SumDOutMin=[]  SumDOutMax=[]  DifferentiatorOutMin=[]  DifferentiatorOutMax=[]  FilterDiffOutCoefMin=[]  FilterDiffOutCoefMax=[]  ReciprocalOutMin=[]  ReciprocalOutMax=[]  SumDenOutMin=[]  SumDenOutMax=[]  SumNumOutMin=[]  SumNumOutMax=[]  DivideOutMin=[]  DivideOutMax=[]  UdiffTsProdOutMin=[]  UdiffTsProdOutMax=[]  NTsProdOutMin=[]  NTsProdOutMax=[]  UintegralTsProdOutMin=[]  UintegralTsProdOutMax=[]  UngainTsProdOutMin=[]  UngainTsProdOutMax=[]  ClampingZeroOutDataTypeStr=Inherit: Inherit via back propagation  ClampingZeroOutMin=[]  ClampingZeroOutMax=[]  FilterDenConstantOutDataTypeStr=Inherit: Inherit via back propagation  FilterDenConstantOutMin=[]  FilterDenConstantOutMax=[]  PCopyOutDataTypeStr=Inherit: Inherit via back propagation  PCopyOutMin=[]  PCopyOutMax=[]  NCopyOutDataTypeStr=Inherit: Inherit via back propagation  NCopyOutMin=[]  NCopyOutMax=[]  IntegratorContinuousStateAttributes=''  IntegratorStateMustResolveToSignalObject=off  IntegratorRTWStateStorageClass=Auto  FilterContinuousStateAttributes=''  FilterStateMustResolveToSignalObject=off  FilterRTWStateStorageClass=Auto  ParallelPVariant=InternalParameters  IdealPVariant=Disabled  IVariant=InternalParameters  DVariant=InternalParameters  IntegratorVariant=Continuous  SatVariant=Disabled  AWVariant=Passthrough  PCopyVariant=Disabled  TRVariant=Disabled  FdbkBlocksVariant=Forward  IdealPFdbkVariant=Disabled  SatFdbkVariant=Disabled  DerivativeFilterVariant=ContFilter  NVariant=InternalParameters  NCopyVariant=Disabled  FilterICVariant=InternalICsFilter  IntegratorICVariant=InternalICs  ExternalResetVariant=Disabled  TRSumVariant=Passthrough  SumFdbkVariant=Disabled  SumVariant=Sum_PID  TsampFilterVariant=InternalTs  TsampNgainVariant=Passthrough  TsampIntegralVariant=Disabled_SignalSpec  ExternalSaturationOutDataTypeStr=Inherit: Same as second input
  tau (body frame) : Outport  VectorParamsAs1DForOutWhenUnconnected=off
  wires:
  eta/1 -> Demux/1  "eta"
  eta set point/1 -> Demux1/1
  Demux/1 -> Sum2/1  "n_vessel"
  Demux1/1 -> Sum2/2  "n_sp"
  Demux/2 -> Sum/1  "e_vessel"
  Demux1/2 -> Sum/2  "e_sp"
  Sum2/1 -> Mux/1
  Sum/1 -> Mux/2
  MATLAB Function/1(y) -> Matrix Multiply/1
  Mux/1 -> Matrix Multiply/2  "error NED frame"
  Step/1 -> Mux2/4, Mux2/3, Mux2/5
  Demux1/3 -> Sum1/2, MATLAB Function1/1(u)  "yaw_sp"
  Sum1/1 -> Yaw PID Controller/1, Mux3/3
  Constant/1 -> Mux/3
  Demux/3 -> MATLAB Function/1(u), Sum1/1  "yaw_vessel"
  Matrix Multiply/1 -> Demux4/1  "error body frame"
  nu/1 -> Sum3/1
  Sum3/1 -> Gain/1  "error body frame"
  nu setpoint/1 -> Matrix Multiply1/2
  MATLAB Function1/1(y) -> Matrix Multiply1/1
  Matrix Multiply1/1 -> Sum3/2
  Integrator/1 -> Gain2/1
  Gain1/1 -> Add/1
  Gain2/1 -> Add/2
  Gain/1 -> Add/3
  Add/1 -> To Workspace/1, Scope/1, Manual Switch/2
  Demux3/1 -> Mux2/1
  Demux3/2 -> Mux2/2
  Demux3/3 -> Mux2/6
  Demux4/1 -> X PID Controller/1, Mux3/1
  Demux4/2 -> Y PID Controller/1, Mux3/2
  Demux4/3 -> Terminator1/1
  Mux3/1 -> Integrator/1, Gain1/1
  Mux2/1 -> tau (body frame)/1
  Manual Switch/1 -> Demux3/1
  X PID Controller/1 -> Mux1/1
  Y PID Controller/1 -> Mux1/2
  Yaw PID Controller/1 -> Mux1/3
  Mux1/1 -> Manual Switch/1

== system part2_MAIN/Simulation 6/Observer ==
  y : Inport
  tau_est : Inport  Port=2
  Demux : Demux  Outputs=2
  EKF : Subsystem
  Memory : Memory  InitialCondition=zeros(3,1)
  Mux : Mux  Inputs=2
  Mux1 : Mux  Inputs=2
  Observer Selector : Constant  Value=observer_type
  Passive Non-Linear : Subsystem
  Subsystem : Subsystem
  Switch : Switch  Criteria=u2 > Threshold  SaturateOnIntegerOverflow=off  InputSameDT=off
  nu_hat : Outport  VectorParamsAs1DForOutWhenUnconnected=off
  eta_hat : Outport  Port=2  VectorParamsAs1DForOutWhenUnconnected=off
  wires:
  y/1 -> EKF/1(y), Passive Non-Linear/1(y)
  tau_est/1 -> Subsystem/1(In1)
  Memory/1 -> EKF/2(U)
  Subsystem/1(Out1) -> Memory/1, Passive Non-Linear/2(tau_est)
  EKF/1(eta_hat) -> Mux/1
  EKF/2(nu_hat) -> Mux/2
  Passive Non-Linear/1(eta_hat) -> Mux1/1
  Passive Non-Linear/2(nu_hat) -> Mux1/2
  Mux1/1 -> Switch/1
  Observer Selector/1 -> Switch/2
  Mux/1 -> Switch/3
  Switch/1 -> Demux/1
  Demux/1 -> eta_hat/1
  Demux/2 -> nu_hat/1

== system part2_MAIN/Simulation 6/Reference Model ==
  note: Af
  note: eta_r
  note: Xref
  note: omega
  note: eta_r - Xref
  note: Gamma
  note: x_ddot
  note: Gamma
  note: X_dot
  note: X
  Add : Sum  Inputs=+--
  Gain : Gain  Gain=Af  Multiplication=Matrix(K*u)
  Gain1 : Gain  Gain=Gamma  Multiplication=Matrix(K*u)
  Gain2 : Gain  Gain=Omega  Multiplication=Matrix(K*u)
  Gain3 : Gain  Gain=Gamma  Multiplication=Matrix(K*u)
  Integrator : Integrator
  Integrator1 : Integrator
  Integrator2 : Integrator
  Scope : Scope  NumInputPorts=2
  Scope1 : Scope
  Scope2 : Scope
  Simulation Selector : Subsystem
  Sum : Sum  Inputs=|+-
  To Workspace : ToWorkspace  VariableName=Reference  SaveFormat=Timeseries  SampleTime=-1
  Set-point : Outport  VectorParamsAs1DForOutWhenUnconnected=off
  nu set point : Outport  Port=2  VectorParamsAs1DForOutWhenUnconnected=off
  wires:
  Integrator/1 -> Gain1/1, Sum/2
  Add/1 -> Scope2/1, Integrator1/1
  Integrator2/1 -> To Workspace/1, Scope/1, Set-point/1, Gain3/1
  Gain1/1 -> Add/1
  Integrator1/1 -> nu set point/1, Scope/2, Integrator2/1, Gain2/1
  Gain/1 -> Integrator/1
  Gain2/1 -> Add/3
  Gain3/1 -> Add/2
  Simulation Selector/1(Out1) -> Scope1/1, Sum/1
  Sum/1 -> Gain/1

== system part2_MAIN/Simulation 6/Thrust Allocation ==
  tau_d : Inport
  0 : MATLAB Function  TreatAsAtomicUnit=on
  1 : MATLAB Function  Commented=on  TreatAsAtomicUnit=on
  Thrust Utilization : MATLAB Function  TreatAsAtomicUnit=on
  To Workspace : ToWorkspace  VariableName=T_u  SaveFormat=Timeseries  SampleTime=-1
  Unwrap : Subsystem
  u : Outport  VectorParamsAs1DForOutWhenUnconnected=off
  alpha [rad] : Outport  Port=2  VectorParamsAs1DForOutWhenUnconnected=off
  wires:
  tau_d/1 -> 1/1(tau_d), 0/1(tau_d)
  0/1(Td) -> Thrust Utilization/1(Td), u/1
  0/2(alpha) -> Unwrap/1(alpha)
  Unwrap/1(alpha [rad]) -> alpha [rad]/1
  Thrust Utilization/1(T_u) -> To Workspace/1

== system part2_MAIN/Simulation 6/Thruster Dynamics ==
  u [N] : Inport
  alpha [rad] : Inport  Port=2
  Constant : Constant  Value=[thrusters(1).xposition, thrusters(2).xposition, thrusters(3).xposition, thrusters(4).xposition, thrusters(5).xposition]
  Constant1 : Constant  Value=zeros(3,1)
  Constant2 : Constant  Value=[thrusters(1).yposition, thrusters(2).yposition, thrusters(3).yposition, thrusters(4).yposition, thrusters(5).yposition]
  Demux : Demux  Outputs=5
  Demux1 : Demux  Outputs=5
  Gain1 : Gain  Gain=1-thrusterfault
  Gain2 : Gain  Gain=1-thrusterfault
  MATLAB Function : MATLAB Function  TreatAsAtomicUnit=on
  Mux1 : Mux  Inputs=2
  Rate Limiter : RateLimiter  RisingSlewLimit=thrusters(1).rate  FallingSlewLimit=-thrusters(1).rate  SampleTimeMode=inherited
  Rate Limiter1 : RateLimiter  RisingSlewLimit=thrusters(2).rate  FallingSlewLimit=-thrusters(2).rate  SampleTimeMode=inherited
  Rate Limiter10 : RateLimiter  RisingSlewLimit=thrusters(4).rotationspeed  FallingSlewLimit=-thrusters(4).rotationspeed  SampleTimeMode=inherited
  Rate Limiter11 : RateLimiter  RisingSlewLimit=thrusters(5).rotationspeed  FallingSlewLimit=-thrusters(5).rotationspeed  SampleTimeMode=inherited
  Rate Limiter2 : RateLimiter  RisingSlewLimit=thrusters(3).rate  FallingSlewLimit=-thrusters(3).rate  SampleTimeMode=inherited
  Rate Limiter4 : RateLimiter  RisingSlewLimit=thrusters(4).rate  FallingSlewLimit=-thrusters(4).rate  SampleTimeMode=inherited
  Rate Limiter5 : RateLimiter  RisingSlewLimit=thrusters(5).rate  FallingSlewLimit=-thrusters(5).rate  SampleTimeMode=inherited
  Rate Limiter8 : RateLimiter  RisingSlewLimit=thrusters(2).rotationspeed  FallingSlewLimit=-thrusters(2).rotationspeed  SampleTimeMode=inherited
  Saturation : Saturate  UpperLimit=thrusters(1).thrust  LowerLimit=-thrusters(1).thrust
  Saturation1 : Saturate  UpperLimit=thrusters(2).thrust  LowerLimit=-thrusters(2).thrust
  Saturation2 : Saturate  UpperLimit=thrusters(3).thrust  LowerLimit=-thrusters(3).thrust
  Saturation4 : Saturate  UpperLimit=thrusters(4).thrust  LowerLimit=-thrusters(4).thrust
  Saturation5 : Saturate  UpperLimit=thrusters(5).thrust  LowerLimit=-thrusters(5).thrust
  Selector4 : Selector  InputPortWidth=6  IndexOptions=Index vector (dialog)  Indices=[1 2 4 5 6 3]  OutputSizes=1
  alpha : Mux  Inputs=5
  u : Mux  Inputs=5
  "Forces (body frame) " : Outport  VectorParamsAs1DForOutWhenUnconnected=off
  wires:
  Rate Limiter2/1 -> u/3
  Saturation/1 -> Rate Limiter/1
  Mux1/1 -> Selector4/1
  Constant1/1 -> Mux1/2
  Saturation4/1 -> Rate Limiter4/1
  Demux/2 -> Saturation1/1
  Saturation1/1 -> Rate Limiter1/1
  Demux/1 -> Saturation/1
  Demux/3 -> Saturation2/1
  Saturation2/1 -> Rate Limiter2/1
  Selector4/1 -> "Forces (body frame) "/1
  Gain1/1 -> u/2
  Rate Limiter1/1 -> Gain1/1
  Rate Limiter/1 -> u/1
  Rate Limiter4/1 -> Gain2/1
  Saturation5/1 -> Rate Limiter5/1
  u [N]/1 -> Demux/1
  alpha [rad]/1 -> Demux1/1
  Constant/1 -> MATLAB Function/3(PosX)
  Constant2/1 -> MATLAB Function/4(PosY)
  u/1 -> MATLAB Function/2(thrust_actual)
  alpha/1 -> MATLAB Function/1(alpha_actual)
  MATLAB Function/1(actual_tau) -> Mux1/1
  Rate Limiter10/1 -> alpha/4
  Demux1/4 -> Rate Limiter10/1
  Demux1/5 -> Rate Limiter11/1
  Rate Limiter11/1 -> alpha/5
  Demux1/1 -> alpha/1
  Gain2/1 -> u/4
  Demux/4 -> Saturation4/1
  Demux/5 -> Saturation5/1
  Rate Limiter5/1 -> u/5
  Demux1/2 -> Rate Limiter8/1
  Rate Limiter8/1 -> alpha/2
  Demux1/3 -> alpha/3

== system part2_MAIN/Simulation 6/Wave ==
  eta : Inport
  waves : Inport  Port=2
  Gain : Gain  Gain=waveforces
  Sum : Sum
  Wave loads (U=0) : marine_hydro/Hydro Library/Wave loads (U=0)  SystemSampleTime=-1  VariantActivationTime=update diagram  AllowFlexibleInterface=on  Latency=0  AutoFrameSizeCalculation=off
  Wave : Outport  VectorParamsAs1DForOutWhenUnconnected=off
  wires:
  eta/1 -> Wave loads (U=0)/1
  waves/1 -> Wave loads (U=0)/2
  Sum/1 -> Gain/1
  Wave loads (U=0)/1 -> Sum/1
  Wave loads (U=0)/2 -> Sum/2
  Gain/1 -> Wave/1

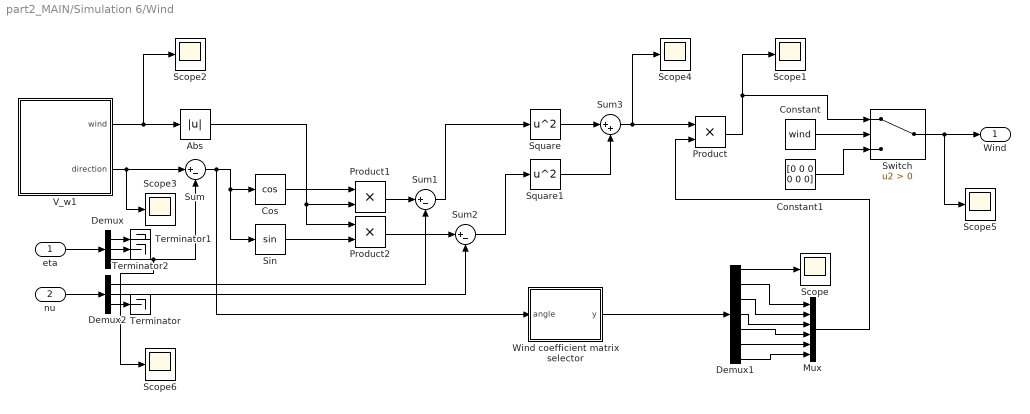
== system part2_MAIN/Simulation 6/Wind ==
  eta : Inport
  nu : Inport  Port=2
  Abs : Abs  SaturateOnIntegerOverflow=off
  Constant : Constant  Value=wind
  Constant1 : Constant  Value=[0 0 0 0 0 0]
  Cos : Trigonometry  Operator=cos
  Demux : Demux  Outputs=3
  Demux1 : Demux  Outputs=7
  Demux2 : Demux  Outputs=3
  Mux : Mux  Inputs=6
  Product : Product
  Product1 : Product
  Product2 : Product
  Scope{,1..6} (7 alike) : Scope
  Sin : Trigonometry
  Square : Math  Operator=square  SignedPower=on
  Square1 : Math  Operator=square  SignedPower=on
  Sum : Sum  Inputs=|+-
  Sum1 : Sum  Inputs=|+-
  Sum2 : Sum  Inputs=|+-
  Sum3 : Sum  Inputs=|++
  Switch : Switch  Criteria=u2 > Threshold  SaturateOnIntegerOverflow=off  InputSameDT=off
  Terminator : Terminator
  Terminator1 : Terminator
  Terminator2 : Terminator
  V_w1 : Subsystem
  Wind coefficient matrix selector : MATLAB Function  TreatAsAtomicUnit=on
  Wind : Outport  VectorParamsAs1DForOutWhenUnconnected=off
  wires:
  V_w1/1(wind) -> Scope2/1, Abs/1
  Abs/1 -> Product2/1, Product1/2
  eta/1 -> Demux/1
  V_w1/2(direction) -> Scope3/1, Sum/1
  Demux/3 -> Scope6/1, Sum/2
  Wind coefficient matrix selector/1(y) -> Demux1/1
  Demux1/1 -> Scope/1
  Demux1/2 -> Mux/1
  Demux1/3 -> Mux/2
  Demux1/4 -> Mux/3
  Demux1/5 -> Mux/4
  Demux1/6 -> Mux/5
  Demux1/7 -> Mux/6
  Product/1 -> Switch/1, Scope1/1
  Mux/1 -> Product/2
  Sum/1 -> Wind coefficient matrix selector/1(angle), Sin/1, Cos/1
  nu/1 -> Demux2/1
  Sin/1 -> Product2/2
  Cos/1 -> Product1/1
  Product1/1 -> Sum1/1
  Product2/1 -> Sum2/1
  Demux2/1 -> Sum1/2
  Demux2/2 -> Sum2/2
  Sum1/1 -> Square/1
  Sum2/1 -> Square1/1
  Sum3/1 -> Scope4/1, Product/1
  Square/1 -> Sum3/1
  Square1/1 -> Sum3/2
  Demux2/3 -> Terminator/1
  Demux/1 -> Terminator1/1
  Demux/2 -> Terminator2/1
  Switch/1 -> Scope5/1, Wind/1
  Constant/1 -> Switch/2
  Constant1/1 -> Switch/3

== system part2_MAIN/Simulation 7/Current (North - East) ==
  note: simulation 2
  note: simulation 1
  eta : Inport
  Constant : Constant
  Constant1 : Constant  Value=[0.5*cos(135); 0.5*sin(135); 0]
  Demux : Demux  Outputs=3
  MATLAB Function : MATLAB Function  TreatAsAtomicUnit=on
  Matrix Multiply : Product  Multiplication=Matrix(*)
  Mux : Mux
  Scope : Scope  NumInputPorts=2
  Scope1 : Scope
  Step : Step  After=0  SampleTime=0
  Subsystem : Subsystem
  Subsystem1 : Subsystem
  Subsystem2 : Subsystem
  Switch : Switch  Criteria=u2 > Threshold  Threshold=1  SaturateOnIntegerOverflow=off  InputSameDT=off
  Switch1 : Switch  Criteria=u2 > Threshold  Threshold=2  SaturateOnIntegerOverflow=off  InputSameDT=off
  Terminator : Terminator
  Terminator1 : Terminator
  Terminator2 : Terminator
  To Workspace : ToWorkspace  VariableName=Current  SaveFormat=Timeseries  SampleTime=-1
  Current1 : Outport  VectorParamsAs1DForOutWhenUnconnected=off
  wires:
  Demux/2 -> Terminator1/1
  MATLAB Function/1(y) -> Matrix Multiply/1
  Switch/1 -> Switch1/3
  Matrix Multiply/1 -> Scope/2, Mux/1
  Subsystem2/1(Out1) -> Switch1/1
  Subsystem/1(Out1) -> Switch/3
  Subsystem1/1(Out1) -> Switch/1
  Demux/1 -> Terminator/1
  Switch1/1 -> Scope/1, To Workspace/1, Matrix Multiply/2
  eta/1 -> Demux/1  "eta"
  Constant/1 -> Switch1/2, Switch/2
  Constant1/1 -> Terminator2/1
  Step/1 -> Mux/3, Mux/2, Mux/4
  Demux/3 -> MATLAB Function/1(u)
  Mux/1 -> Scope1/1, Current1/1

== system part2_MAIN/Simulation 7/DP Controller ==
  note: PID controller
  note: Velocity
  note: Position
  nu : Inport
  eta : Inport  Port=2
  eta set point : Inport  Port=3
  nu setpoint : Inport  Port=4
  Add : Sum  Inputs=+++
  Constant : Constant  Value=0
  Demux{,1,3..4} (4 alike) : Demux  Outputs=3
  Gain : Gain  Gain=Kd
  Gain1 : Gain  Gain=Kp
  Gain2 : Gain  Gain=Ki
  Integrator : Integrator
  MATLAB Function : MATLAB Function  TreatAsAtomicUnit=on
  MATLAB Function1 : MATLAB Function  TreatAsAtomicUnit=on
  Matrix Multiply : Product  Multiplication=Matrix(*)
  Matrix Multiply1 : Product  Multiplication=Matrix(*)
  Mux : Mux  Inputs=3
  Mux2 : Mux  Inputs=6
  Mux3 : Mux  Inputs=3
  Scope : Scope
  Step : Step  After=0  SampleTime=0
  Sum{,1..3} (4 alike) : Sum  Inputs=|-+
  Terminator1 : Terminator
  To Workspace : ToWorkspace  VariableName=simout2  SaveFormat=Timeseries  SampleTime=-1
  tau (body frame) : Outport  VectorParamsAs1DForOutWhenUnconnected=off
  wires:
  eta/1 -> Demux/1  "eta"
  eta set point/1 -> Demux1/1
  Demux/1 -> Sum2/1  "n_vessel"
  Demux1/1 -> Sum2/2  "n_sp"
  Demux/2 -> Sum/1  "e_vessel"
  Demux1/2 -> Sum/2  "e_sp"
  Sum2/1 -> Mux/1
  Sum/1 -> Mux/2
  MATLAB Function/1(y) -> Matrix Multiply/1
  Mux/1 -> Matrix Multiply/2  "error NED frame"
  Step/1 -> Mux2/4, Mux2/3, Mux2/5
  Demux1/3 -> Sum1/2, MATLAB Function1/1(u)  "yaw_sp"
  Sum1/1 -> Mux3/3
  Constant/1 -> Mux/3
  Demux/3 -> MATLAB Function/1(u), Sum1/1  "yaw_vessel"
  Matrix Multiply/1 -> Demux4/1  "error body frame"
  nu/1 -> Sum3/1
  Sum3/1 -> Gain/1  "error body frame"
  nu setpoint/1 -> Matrix Multiply1/2
  MATLAB Function1/1(y) -> Matrix Multiply1/1
  Matrix Multiply1/1 -> Sum3/2
  Integrator/1 -> Gain2/1
  Gain1/1 -> Add/1
  Gain2/1 -> Add/2
  Gain/1 -> Add/3
  Demux3/1 -> Mux2/1
  Demux3/2 -> Mux2/2
  Demux3/3 -> Mux2/6
  Demux4/1 -> Mux3/1
  Demux4/2 -> Mux3/2
  Demux4/3 -> Terminator1/1
  Mux3/1 -> Integrator/1, Gain1/1
  Mux2/1 -> tau (body frame)/1
  Add/1 -> To Workspace/1, Scope/1, Demux3/1

== system part2_MAIN/Simulation 7/Observer ==
  y : Inport
  tau_est : Inport  Port=2
  Demux : Demux  Outputs=2
  EKF : Subsystem
  Memory : Memory  InitialCondition=zeros(3,1)
  Memory2 : Memory  InitialCondition=zeros(3,1)
  Mux : Mux  Inputs=2
  Mux1 : Mux  Inputs=2
  Observer Selector : Constant  Value=observer_type
  Passive Non-Linear : Subsystem
  Subsystem : Subsystem
  Switch : Switch  Criteria=u2 > Threshold  SaturateOnIntegerOverflow=off  InputSameDT=off
  nu_hat : Outport  VectorParamsAs1DForOutWhenUnconnected=off
  eta_hat : Outport  Port=2  VectorParamsAs1DForOutWhenUnconnected=off
  wires:
  tau_est/1 -> Subsystem/1(In1)
  Memory/1 -> EKF/2(U)
  Subsystem/1(Out1) -> Memory/1, Memory2/1
  EKF/1(eta_hat) -> Mux/1
  EKF/2(nu_hat) -> Mux/2
  Passive Non-Linear/1(eta_hat) -> Mux1/1
  Passive Non-Linear/2(nu_hat) -> Mux1/2
  Mux1/1 -> Switch/1
  Observer Selector/1 -> Switch/2
  Mux/1 -> Switch/3
  Switch/1 -> Demux/1
  Demux/1 -> eta_hat/1
  Demux/2 -> nu_hat/1
  y/1 -> EKF/1(y), Passive Non-Linear/1(y)
  Memory2/1 -> Passive Non-Linear/2(tau_est)

== system part2_MAIN/Simulation 7/Reference Model ==
  note: Af
  note: eta_r
  note: Xref
  note: omega
  note: eta_r - Xref
  note: Gamma
  note: x_ddot
  note: Gamma
  note: X_dot
  note: X
  Add : Sum  Inputs=+--
  Gain : Gain  Gain=Af  Multiplication=Matrix(K*u)
  Gain1 : Gain  Gain=Gamma  Multiplication=Matrix(K*u)
  Gain2 : Gain  Gain=Omega  Multiplication=Matrix(K*u)
  Gain3 : Gain  Gain=Gamma  Multiplication=Matrix(K*u)
  Integrator : Integrator
  Integrator1 : Integrator
  Integrator2 : Integrator
  Scope : Scope  NumInputPorts=2
  Scope1 : Scope
  Scope2 : Scope
  Simulation Selector : Subsystem
  Sum : Sum  Inputs=|+-
  To Workspace : ToWorkspace  VariableName=Reference  SaveFormat=Timeseries  SampleTime=-1
  Set-point : Outport  VectorParamsAs1DForOutWhenUnconnected=off
  nu set point : Outport  Port=2  VectorParamsAs1DForOutWhenUnconnected=off
  wires:
  Integrator/1 -> Gain1/1, Sum/2
  Add/1 -> Scope2/1, Integrator1/1
  Integrator2/1 -> To Workspace/1, Scope/1, Set-point/1, Gain3/1
  Gain1/1 -> Add/1
  Integrator1/1 -> nu set point/1, Scope/2, Integrator2/1, Gain2/1
  Gain/1 -> Integrator/1
  Gain2/1 -> Add/3
  Gain3/1 -> Add/2
  Simulation Selector/1(Out1) -> Scope1/1, Sum/1
  Sum/1 -> Gain/1

== system part2_MAIN/Simulation 7/Thrust Allocation ==
  tau_d : Inport
  0 : MATLAB Function  TreatAsAtomicUnit=on
  1 : MATLAB Function  Commented=on  TreatAsAtomicUnit=on
  Constant : Constant  Value=thruster_type
  Switch : Switch  Criteria=u2 > Threshold  SaturateOnIntegerOverflow=off  InputSameDT=off
  Switch1 : Switch  Criteria=u2 > Threshold  SaturateOnIntegerOverflow=off  InputSameDT=off
  Unwrap : Subsystem
  Unwrap1 : Subsystem
  u : Outport  VectorParamsAs1DForOutWhenUnconnected=off
  alpha [rad] : Outport  Port=2  VectorParamsAs1DForOutWhenUnconnected=off
  wires:
  tau_d/1 -> 1/1(tau_d), 0/1(tau_d)
  1/2(alpha) -> Unwrap/1(alpha)
  0/2(alpha) -> Unwrap1/1(alpha)
  1/1(Td) -> Switch/1
  Constant/1 -> Switch1/2, Switch/2
  0/1(Td) -> Switch/3
  Unwrap/1(alpha [rad]) -> Switch1/1
  Unwrap1/1(alpha [rad]) -> Switch1/3
  Switch/1 -> u/1
  Switch1/1 -> alpha [rad]/1

== system part2_MAIN/Simulation 7/Thruster Dynamics ==
  u [N] : Inport
  alpha [rad] : Inport  Port=2
  Constant : Constant  Value=[thrusters(1).xposition, thrusters(2).xposition, thrusters(3).xposition, thrusters(4).xposition, thrusters(5).xposition]
  Constant1 : Constant  Value=zeros(3,1)
  Constant2 : Constant  Value=[thrusters(1).yposition, thrusters(2).yposition, thrusters(3).yposition, thrusters(4).yposition, thrusters(5).yposition]
  Demux : Demux  Outputs=5
  Demux1 : Demux  Outputs=5
  Gain1 : Gain  Gain=1-thrusterfault
  Gain2 : Gain  Gain=1-thrusterfault
  MATLAB Function : MATLAB Function  TreatAsAtomicUnit=on
  Mux1 : Mux  Inputs=2
  Rate Limiter : RateLimiter  RisingSlewLimit=thrusters(1).rate  FallingSlewLimit=-thrusters(1).rate  SampleTimeMode=inherited
  Rate Limiter1 : RateLimiter  RisingSlewLimit=thrusters(2).rate  FallingSlewLimit=-thrusters(2).rate  SampleTimeMode=inherited
  Rate Limiter10 : RateLimiter  RisingSlewLimit=thrusters(4).rotationspeed  FallingSlewLimit=-thrusters(4).rotationspeed  SampleTimeMode=inherited
  Rate Limiter11 : RateLimiter  RisingSlewLimit=thrusters(5).rotationspeed  FallingSlewLimit=-thrusters(5).rotationspeed  SampleTimeMode=inherited
  Rate Limiter2 : RateLimiter  RisingSlewLimit=thrusters(3).rate  FallingSlewLimit=-thrusters(3).rate  SampleTimeMode=inherited
  Rate Limiter4 : RateLimiter  RisingSlewLimit=thrusters(4).rate  FallingSlewLimit=-thrusters(4).rate  SampleTimeMode=inherited
  Rate Limiter5 : RateLimiter  RisingSlewLimit=thrusters(5).rate  FallingSlewLimit=-thrusters(5).rate  SampleTimeMode=inherited
  Rate Limiter8 : RateLimiter  RisingSlewLimit=thrusters(2).rotationspeed  FallingSlewLimit=-thrusters(2).rotationspeed  SampleTimeMode=inherited
  Saturation : Saturate  UpperLimit=thrusters(1).thrust  LowerLimit=-thrusters(1).thrust
  Saturation1 : Saturate  UpperLimit=thrusters(2).thrust  LowerLimit=-thrusters(2).thrust
  Saturation2 : Saturate  UpperLimit=thrusters(3).thrust  LowerLimit=-thrusters(3).thrust
  Saturation4 : Saturate  UpperLimit=thrusters(4).thrust  LowerLimit=-thrusters(4).thrust
  Saturation5 : Saturate  UpperLimit=thrusters(5).thrust  LowerLimit=-thrusters(5).thrust
  Selector4 : Selector  InputPortWidth=6  IndexOptions=Index vector (dialog)  Indices=[1 2 4 5 6 3]  OutputSizes=1
  alpha : Mux  Inputs=5
  u : Mux  Inputs=5
  "Forces (body frame) " : Outport  VectorParamsAs1DForOutWhenUnconnected=off
  wires:
  Rate Limiter2/1 -> u/3
  Saturation/1 -> Rate Limiter/1
  Mux1/1 -> Selector4/1
  Constant1/1 -> Mux1/2
  Saturation4/1 -> Rate Limiter4/1
  Demux/2 -> Saturation1/1
  Saturation1/1 -> Rate Limiter1/1
  Demux/1 -> Saturation/1
  Demux/3 -> Saturation2/1
  Saturation2/1 -> Rate Limiter2/1
  Selector4/1 -> "Forces (body frame) "/1
  Gain1/1 -> u/2
  Rate Limiter1/1 -> Gain1/1
  Rate Limiter/1 -> u/1
  Rate Limiter4/1 -> Gain2/1
  Saturation5/1 -> Rate Limiter5/1
  u [N]/1 -> Demux/1
  alpha [rad]/1 -> Demux1/1
  Constant/1 -> MATLAB Function/3(PosX)
  Constant2/1 -> MATLAB Function/4(PosY)
  u/1 -> MATLAB Function/2(thrust_actual)
  alpha/1 -> MATLAB Function/1(alpha_actual)
  MATLAB Function/1(actual_tau) -> Mux1/1
  Rate Limiter10/1 -> alpha/4
  Demux1/4 -> Rate Limiter10/1
  Demux1/5 -> Rate Limiter11/1
  Rate Limiter11/1 -> alpha/5
  Demux1/1 -> alpha/1
  Gain2/1 -> u/4
  Demux/4 -> Saturation4/1
  Demux/5 -> Saturation5/1
  Rate Limiter5/1 -> u/5
  Demux1/2 -> Rate Limiter8/1
  Rate Limiter8/1 -> alpha/2
  Demux1/3 -> alpha/3
